simulink model "template_CM_CS_lookup_with_comments_to_Mr_Fs_calc"  (R2016a)
settings: Solver=ode45  StartTime=0.0  StopTime=10.0  RelTol=1e-3
values from neighbouring files (symbols this model uses):
  beta_array = [0 0.0872664625997 0.174532925199 0.261799387799 0.349065850399 0.436332312999 0.523598775598 0.698131700798 0.872664625997 1.0471975512 1.2217304764 1.3962634016 ... (13 elements, 1x13)]    [CQ_CT_maps.mat]
  CQ_entries = [0.00463492513935 0.0049015417371 0.00516815833485 0.00555696036228 0.0059457623897 0.00611397686765 0.00628219134561 0.012914252991 0.0255245334589 0.0349006692545 0.0430149587943 0.0524658396931 ... (507 elements, 39x13)]    [CQ_CT_maps.mat]
  CT_entries = [0.0686211548678 0.0728422059393 0.0770632570108 0.0836290674204 0.09019487783 0.0932108047116 0.0962267315932 0.135717354129 0.192838891055 0.239446349533 0.288110808378 0.351656989082 ... (507 elements, 39x13)]    [CQ_CT_maps.mat]
  lambda_array = [0 0.25 0.5 0.75 1 1.25 1.5 2 2.5 3 3.5 4 ... (39 elements, 39x1)]    [CQ_CT_maps.mat]
settings Model: Creator=schulte  LastModifiedBy=schulte
settings DataIOCC: LimitDataPoints=on  SaveFormat=Array
settings DebuggingCC: SolverPrmCheckMsg=warning
settings HardwareCC: ProdBitPerPointer=32  ProdLargestAtomicFloat=None  ProdIntDivRoundTo=Undefined  ProdEndianess=Unspecified  ProdWordSize=32  ProdHWDeviceType=32-bit Generic
settings ModelReferenceCC: PropagateSignalLabelsOutOfModel=off
settings ConfigComp: CovModelRefEnable=Off  CovSFcnEnable=off

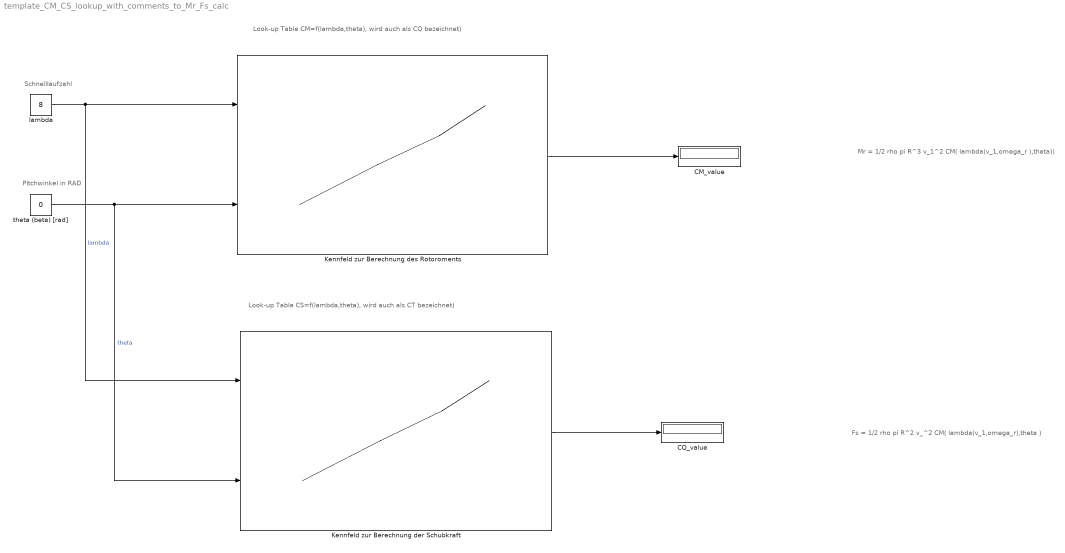
== system template_CM_CS_lookup_with_comments_to_Mr_Fs_calc ==
  note: Fs = 1/2 rho pi R^2 v_^2 CM( lambda(v_1,omega_r),theta )
  note: Mr = 1/2 rho pi R^3 v_1^2 CM( lambda(v_1,omega_r ),theta))
  note: Pitchwinkel in RAD
  note: Schnelllaufzahl
  note: Look-up Table CM=f(lambda,theta), wird auch als CQ bezeichnet)
  note: Look-up Table CS=f(lambda,theta), wird auch als CT bezeichnet)
  CM_value : Display
  CQ_value : Display
  Kennfeld zur Berechnung der Schubkraft : Lookup_n-D  BreakpointsForDimension1=lambda_array  BreakpointsForDimension2=beta_array  Table=CT_entries  InternalRulePriority=Speed  RndMeth=Simplest  InputSameDT=on
  Kennfeld zur Berechnung des Rotoroments : Lookup_n-D  BreakpointsForDimension1=lambda_array  BreakpointsForDimension2=beta_array  Table=CQ_entries  InternalRulePriority=Speed  RndMeth=Simplest  InputSameDT=on
  lambda : Constant  Value=8
  theta (beta) [rad] : Constant  Value=0
  wires:
  lambda/1 -> Kennfeld zur Berechnung der Schubkraft/1, Kennfeld zur Berechnung des Rotoroments/1  "lambda"
  theta (beta) [rad]/1 -> Kennfeld zur Berechnung der Schubkraft/2, Kennfeld zur Berechnung des Rotoroments/2  "theta"
  Kennfeld zur Berechnung des Rotoroments/1 -> CM_value/1
  Kennfeld zur Berechnung der Schubkraft/1 -> CQ_value/1
